simulink model "openMHA_test_db_ar_gaintable"  (R2020b)
settings: Solver=VariableStepAuto  StartTime=0.0  StopTime=stop_time  RelTol=1e-3
InitFcn:
  | initCallback
StopFcn:
  | stopCallback
values from neighbouring files (symbols this model uses):
  buf_a = 65.*ones(num_bands,1)    [test_FFT_to_gain_init.m]    (also in test_db_ar_gaintable_init.m)
  num_bands = 8    [test_FFT_to_gain_init.m]    (also in test_db_ar_gaintable_init.m = 2)
  table_length = length(gtdata)    [test_FFT_to_gain_init.m]    (also in test_db_ar_gaintable_init.m)
  X_high = 93    [test_FFT_to_gain_init.m]    (also in test_db_ar_gaintable_init.m)
undefined symbols (not defined in the file or in its folder): xIn
libraries: dspsrcs4 x13, FPGA_Open_Speech_Tools x4, simulink x4
settings Model: PacingRate=200  Creator=t96f346  LastModifiedBy=wickh

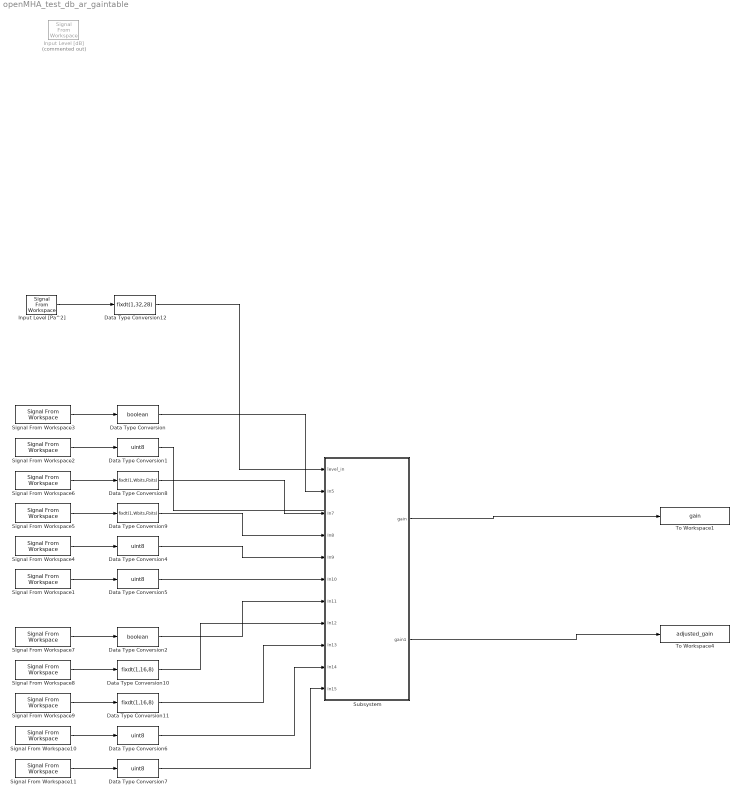
== system openMHA_test_db_ar_gaintable ==
  Data Type Conversion : DataTypeConversion  OutDataTypeStr=boolean
  Data Type Conversion{1,4..7} (5 alike) : DataTypeConversion  OutDataTypeStr=uint8
  Data Type Conversion10 : DataTypeConversion  OutDataTypeStr=fixdt(1,16,8)
  Data Type Conversion11 : DataTypeConversion  OutDataTypeStr=fixdt(1,16,8)
  Data Type Conversion12 : DataTypeConversion  OutDataTypeStr=fixdt(1,32,28)
  Data Type Conversion2 : DataTypeConversion  OutDataTypeStr=boolean
  Data Type Conversion8 : DataTypeConversion  OutDataTypeStr=fixdt(1,Wbits,Fbits)
  Data Type Conversion9 : DataTypeConversion  OutDataTypeStr=fixdt(1,Wbits,Fbits)
  Input Level [Pa^2] : dspsrcs4/Signal From Workspace  X=level_in  Ts=1  nsamps=1  OutputAfterFinalValue=Setting to zero  ignoreOrWarnInputAndFrameLengths=off  OutputFrames=off
  Input Level [dB] : dspsrcs4/Signal From Workspace  Commented=on  X=Lst  Ts=1  nsamps=1  OutputAfterFinalValue=Setting to zero  ignoreOrWarnInputAndFrameLengths=off  OutputFrames=off
  Signal From Workspace1 : dspsrcs4/Signal From Workspace  X=write_addr_r  Ts=1  nsamps=1  OutputAfterFinalValue=Setting to zero  ignoreOrWarnInputAndFrameLengths=off  OutputFrames=off
  Signal From Workspace10 : dspsrcs4/Signal From Workspace  X=write_addr_vy_low  Ts=1  nsamps=1  OutputAfterFinalValue=Setting to zero  ignoreOrWarnInputAndFrameLengths=off  OutputFrames=off
  Signal From Workspace11 : dspsrcs4/Signal From Workspace  X=write_addr_vy_high  Ts=1  nsamps=1  OutputAfterFinalValue=Setting to zero  ignoreOrWarnInputAndFrameLengths=off  OutputFrames=off
  Signal From Workspace2 : dspsrcs4/Signal From Workspace  X=band_num  Ts=1  nsamps=1  OutputAfterFinalValue=Setting to zero  ignoreOrWarnInputAndFrameLengths=off  OutputFrames=off
  Signal From Workspace3 : dspsrcs4/Signal From Workspace  X=write_en_ar  Ts=1  nsamps=1  OutputAfterFinalValue=Setting to zero  ignoreOrWarnInputAndFrameLengths=off  OutputFrames=off
  Signal From Workspace4 : dspsrcs4/Signal From Workspace  X=write_addr_a  Ts=1  nsamps=1  OutputAfterFinalValue=Setting to zero  ignoreOrWarnInputAndFrameLengths=off  OutputFrames=off
  Signal From Workspace5 : dspsrcs4/Signal From Workspace  X=write_data_r  Ts=1  nsamps=1  OutputAfterFinalValue=Setting to zero  ignoreOrWarnInputAndFrameLengths=off  OutputFrames=off
  Signal From Workspace6 : dspsrcs4/Signal From Workspace  X=write_data_a  Ts=1  nsamps=1  OutputAfterFinalValue=Setting to zero  ignoreOrWarnInputAndFrameLengths=off  OutputFrames=off
  Signal From Workspace7 : dspsrcs4/Signal From Workspace  X=write_en_vy  Ts=1  nsamps=1  OutputAfterFinalValue=Setting to zero  ignoreOrWarnInputAndFrameLengths=off  OutputFrames=off
  Signal From Workspace8 : dspsrcs4/Signal From Workspace  X=write_data_vy_low  Ts=1  nsamps=1  OutputAfterFinalValue=Setting to zero  ignoreOrWarnInputAndFrameLengths=off  OutputFrames=off
  Signal From Workspace9 : dspsrcs4/Signal From Workspace  X=write_data_vy_high  Ts=1  nsamps=1  OutputAfterFinalValue=Setting to zero  ignoreOrWarnInputAndFrameLengths=off  OutputFrames=off
  Subsystem : Subsystem
  To Workspace1 : ToWorkspace  VariableName=gain  SampleTime=-1
      settings: Save2DSignal=2-D array (concatenate along first dimension)
  To Workspace4 : ToWorkspace  VariableName=adjusted_gain  SampleTime=-1
      settings: Save2DSignal=2-D array (concatenate along first dimension)
  wires:
  Signal From Workspace2/1 -> Data Type Conversion1/1
  Signal From Workspace3/1 -> Data Type Conversion/1
  Signal From Workspace7/1 -> Data Type Conversion2/1
  Signal From Workspace8/1 -> Data Type Conversion10/1
  Signal From Workspace9/1 -> Data Type Conversion11/1
  Signal From Workspace10/1 -> Data Type Conversion6/1
  Signal From Workspace11/1 -> Data Type Conversion7/1
  Signal From Workspace6/1 -> Data Type Conversion8/1
  Signal From Workspace5/1 -> Data Type Conversion9/1
  Signal From Workspace4/1 -> Data Type Conversion4/1
  Signal From Workspace1/1 -> Data Type Conversion5/1
  Input Level [Pa^2]/1 -> Data Type Conversion12/1
  Data Type Conversion12/1 -> Subsystem/1(level_in)
  Data Type Conversion/1 -> Subsystem/2(In5)
  Data Type Conversion1/1 -> ?
  Data Type Conversion8/1 -> Subsystem/3(In7)
  Data Type Conversion9/1 -> Subsystem/4(In8)
  Data Type Conversion4/1 -> Subsystem/5(In9)
  Data Type Conversion5/1 -> Subsystem/6(In10)
  Data Type Conversion2/1 -> Subsystem/7(In11)
  Data Type Conversion10/1 -> Subsystem/8(In12)
  Data Type Conversion11/1 -> Subsystem/9(In13)
  Data Type Conversion6/1 -> Subsystem/10(In14)
  Data Type Conversion7/1 -> Subsystem/11(In15)
  Subsystem/1(gain) -> To Workspace1/1
  Subsystem/2(gain1) -> To Workspace4/1

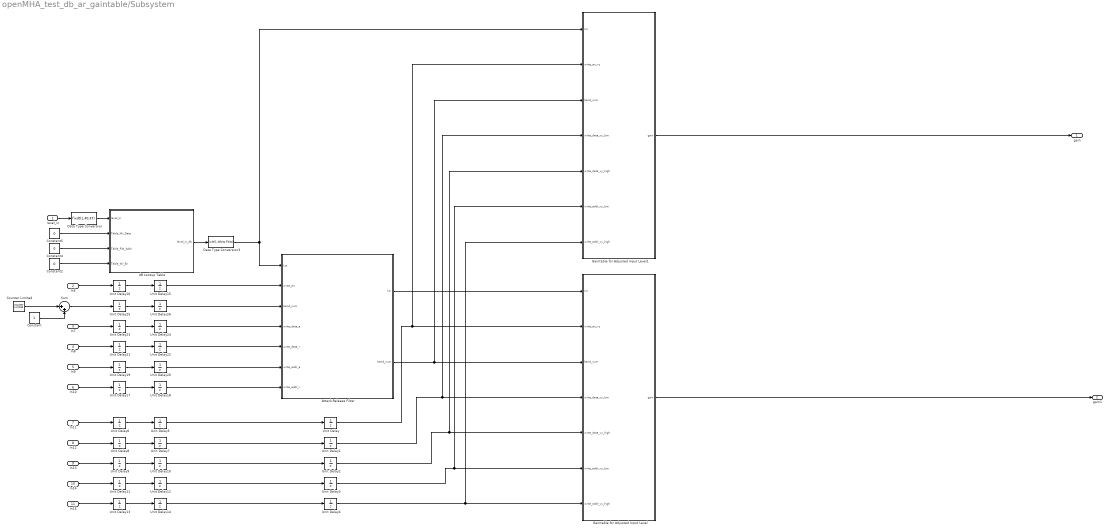
== system openMHA_test_db_ar_gaintable/Subsystem ==
  level_in : Inport
  In5 : Inport  Port=2
  In7 : Inport  Port=3
  In8 : Inport  Port=4
  In9 : Inport  Port=5
  In10 : Inport  Port=6
  In11 : Inport  Port=7
  In12 : Inport  Port=8
  In13 : Inport  Port=9
  In14 : Inport  Port=10
  In15 : Inport  Port=11
  Attack-Release Filter : Subsystem
  Constant : Constant
  Constant2 : Constant  Value=0  OutDataTypeStr=boolean  SampleTime=-1
  Constant4 : Constant  Value=0  OutDataTypeStr=uint16  SampleTime=-1
  Constant5 : Constant  Value=0  OutDataTypeStr=fixdt(1,40,32)  SampleTime=-1
  Counter Limited : simulink/Sources/Counter Limited  uplimit=num_bands-1  tsamp=-1
  Data Type Conversion : DataTypeConversion  OutDataTypeStr=fixdt(1,40,37)
  Data Type Conversion3 : DataTypeConversion  OutDataTypeStr=fixdt(1,Wbits,Fbits)
  Gaintable for Adjusted Input Level : Subsystem
  Gaintable for Adjusted Input Level1 : Subsystem
  Sum : Sum  Inputs=|++
  Unit Delay{,1..3,5..12,15..16,19..26} (22 alike) : UnitDelay  SampleTime=-1  HasFrameUpgradeWarning=on
  Unit Delay{4,13..14,17..18} (5 alike) : UnitDelay  InitialCondition=1  SampleTime=-1  HasFrameUpgradeWarning=on
  dB Lookup Table : Subsystem
  gain : Outport
  gain1 : Outport  Port=2
  wires:
  Unit Delay5/1 -> Unit Delay/1
  Unit Delay24/1 -> Attack-Release Filter/4(write_data_a)
  In8/1 -> Unit Delay21/1
  Unit Delay/1 -> Gaintable for Adjusted Input Level1/2(write_en_vy), Gaintable for Adjusted Input Level/2(write_en_vy)
  In12/1 -> Unit Delay8/1
  Unit Delay2/1 -> Gaintable for Adjusted Input Level1/5(write_data_vy_high), Gaintable for Adjusted Input Level/5(write_data_vy_high)
  Data Type Conversion3/1 -> Attack-Release Filter/1(Lst), Gaintable for Adjusted Input Level1/1(Lin)
  Unit Delay4/1 -> Gaintable for Adjusted Input Level1/7(write_addr_vy_high), Gaintable for Adjusted Input Level/7(write_addr_vy_high)
  Unit Delay26/1 -> Attack-Release Filter/3(band_num)
  In10/1 -> Unit Delay17/1
  In9/1 -> Unit Delay19/1
  Unit Delay17/1 -> Unit Delay18/1
  Attack-Release Filter/1(Lin) -> Gaintable for Adjusted Input Level/1(Lin)
  Unit Delay9/1 -> Unit Delay10/1
  Attack-Release Filter/2("band_num ") -> Gaintable for Adjusted Input Level1/3(band_num), Gaintable for Adjusted Input Level/3(band_num)
  Unit Delay1/1 -> Gaintable for Adjusted Input Level1/4(write_data_vy_low), Gaintable for Adjusted Input Level/4(write_data_vy_low)
  In13/1 -> Unit Delay9/1
  Unit Delay13/1 -> Unit Delay14/1
  Unit Delay11/1 -> Unit Delay12/1
  Unit Delay6/1 -> Unit Delay5/1
  Unit Delay12/1 -> Unit Delay3/1
  Constant2/1 -> dB Lookup Table/4(Table_Wr_En)
  Unit Delay10/1 -> Unit Delay2/1
  Unit Delay7/1 -> Unit Delay1/1
  Unit Delay3/1 -> Gaintable for Adjusted Input Level1/6(write_addr_vy_low), Gaintable for Adjusted Input Level/6(write_addr_vy_low)
  Unit Delay15/1 -> Attack-Release Filter/2(write_en)
  In14/1 -> Unit Delay11/1
  Unit Delay20/1 -> Attack-Release Filter/6(write_addr_a)
  dB Lookup Table/1(level_in_db) -> Data Type Conversion3/1
  Unit Delay18/1 -> Attack-Release Filter/7(write_addr_r)
  In5/1 -> Unit Delay16/1
  Unit Delay16/1 -> Unit Delay15/1
  Unit Delay8/1 -> Unit Delay7/1
  In7/1 -> Unit Delay23/1
  Unit Delay19/1 -> Unit Delay20/1
  Sum/1 -> Unit Delay25/1
  Unit Delay21/1 -> Unit Delay22/1
  Unit Delay25/1 -> Unit Delay26/1
  In11/1 -> Unit Delay6/1
  Unit Delay22/1 -> Attack-Release Filter/5(write_data_r)
  Unit Delay23/1 -> Unit Delay24/1
  Gaintable for Adjusted Input Level1/1(gain) -> gain/1
  Unit Delay14/1 -> Unit Delay4/1
  In15/1 -> Unit Delay13/1
  Constant5/1 -> dB Lookup Table/2(Table_Wr_Data)
  Gaintable for Adjusted Input Level/1(gain) -> gain1/1
  Constant4/1 -> dB Lookup Table/3(Table_RW_Addr)
  level_in/1 -> Data Type Conversion/1
  Data Type Conversion/1 -> dB Lookup Table/1(level_in)
  Counter Limited/1 -> Sum/1
  Constant/1 -> Sum/2

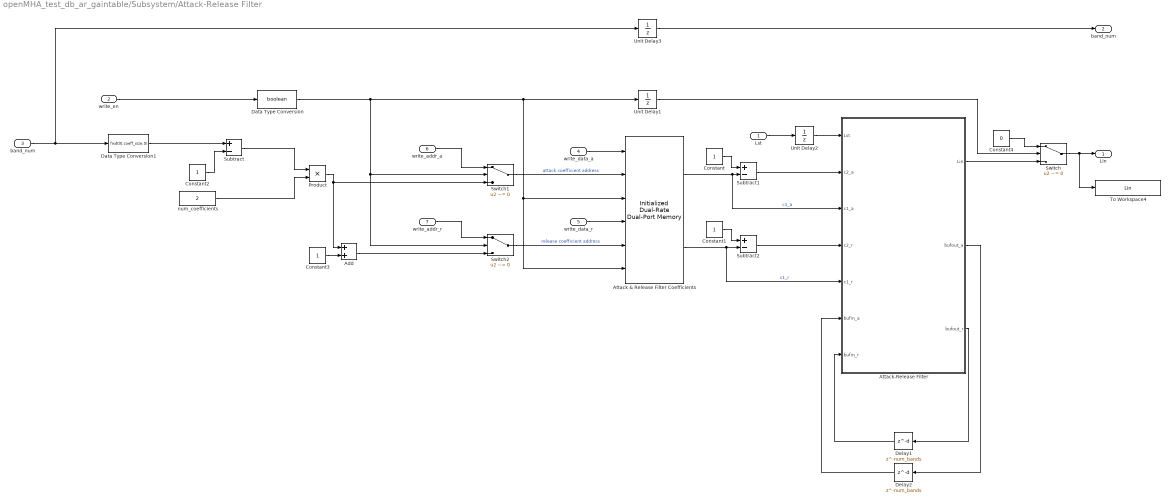
== system openMHA_test_db_ar_gaintable/Subsystem/Attack-Release Filter ==
  Lst : Inport
  write_en : Inport  Port=2
  band_num : Inport  Port=3
  write_data_a : Inport  Port=4
  write_data_r : Inport  Port=5
  write_addr_a : Inport  Port=6
  write_addr_r : Inport  Port=7
  Add : Sum
  Attack & Release Filter Coefficients : FPGA_Open_Speech_Tools/Initialized Dual-Rate Dual-Port Memory  ram_size=coeff_size  Table_Init=ar_coeffs
      settings: SourceProductName=FPGA Open Speech Tools
  Attack-Release Filter : Subsystem
  Constant : Constant  OutDataTypeStr=fixdt(1,Wbits,Fbits)  SampleTime=-1
  Constant1 : Constant  OutDataTypeStr=fixdt(1,Wbits,Fbits)  SampleTime=-1
  Constant2 : Constant  OutDataTypeStr=fixdt(0,coeff_size,0)  SampleTime=-1
  Constant3 : Constant  OutDataTypeStr=uint8  SampleTime=-1
  Constant4 : Constant  Value=0  OutDataTypeStr=fixdt(1,Wbits,Fbits)  SampleTime=-1
  Data Type Conversion : DataTypeConversion  OutDataTypeStr=boolean
  Data Type Conversion1 : DataTypeConversion  OutDataTypeStr=fixdt(0,coeff_size,0)
  Delay1 : Delay  DelayLength=num_bands  InitialCondition=buf_a  UseCircularBuffer=on
  Delay2 : Delay  DelayLength=num_bands  InitialCondition=buf_a  UseCircularBuffer=on
  Product : Product  OutDataTypeStr=fixdt(0,coeff_size,0)
  Subtract : Sum  Inputs=+-  OutDataTypeStr=fixdt(0,coeff_size,0)
  Subtract1 : Sum  Inputs=+-  OutDataTypeStr=fixdt(1,Wbits,Fbits)
  Subtract2 : Sum  Inputs=+-  OutDataTypeStr=fixdt(1,Wbits,Fbits)
  Switch : Switch  Criteria=u2 ~= 0  OutDataTypeStr=fixdt(1,Wbits,Fbits)
  Switch1 : Switch  Criteria=u2 ~= 0  OutDataTypeStr=Inherit: Inherit via back propagation
  Switch2 : Switch  Criteria=u2 ~= 0  OutDataTypeStr=uint8
  To Workspace4 : ToWorkspace  VariableName=Lin  SampleTime=-1
      settings: Save2DSignal=2-D array (concatenate along first dimension)
  Unit Delay1 : UnitDelay  SampleTime=-1  HasFrameUpgradeWarning=on
  Unit Delay2 : UnitDelay  InitialCondition=65  SampleTime=-1  HasFrameUpgradeWarning=on
  Unit Delay3 : UnitDelay  SampleTime=-1  HasFrameUpgradeWarning=on
  num_coefficients : Constant  Value=2  OutDataTypeStr=uint8  SampleTime=-1
  Lin : Outport
  "band_num " : Outport  Port=2
  wires:
  Delay2/1 -> Attack-Release Filter/6(bufin_a)
  write_data_a/1 -> Attack & Release Filter Coefficients/1
  Switch1/1 -> Attack & Release Filter Coefficients/2  "attack coefficient address"
  Switch2/1 -> Attack & Release Filter Coefficients/5  "release coefficient address"
  write_data_r/1 -> Attack & Release Filter Coefficients/4
  Attack-Release Filter/3(bufout_r) -> Delay1/1
  Unit Delay2/1 -> Attack-Release Filter/1(Lst)
  Unit Delay1/1 -> Switch/2
  Lst/1 -> Unit Delay2/1
  Constant1/1 -> Subtract2/1
  Constant/1 -> Subtract1/1
  Switch/1 -> To Workspace4/1, Lin/1
  Attack-Release Filter/1(Lin) -> Switch/3
  Attack-Release Filter/2(bufout_a) -> Delay2/1
  Data Type Conversion/1 -> Unit Delay1/1, Attack & Release Filter Coefficients/3, Attack & Release Filter Coefficients/6, Switch1/2, Switch2/2
  band_num/1 -> Unit Delay3/1, Data Type Conversion1/1
  Constant4/1 -> Switch/1
  write_addr_r/1 -> Switch2/1
  write_en/1 -> Data Type Conversion/1
  Product/1 -> Switch1/3, Add/1
  Delay1/1 -> Attack-Release Filter/7(bufin_r)
  Constant3/1 -> Add/2
  Subtract2/1 -> Attack-Release Filter/4(c2_r)
  Data Type Conversion1/1 -> Subtract/1
  Subtract1/1 -> Attack-Release Filter/2(c2_a)
  write_addr_a/1 -> Switch1/1
  Subtract/1 -> Product/1
  num_coefficients/1 -> Product/2
  Attack & Release Filter Coefficients/2 -> Attack-Release Filter/5(c1_r), Subtract2/2  "c1_r"
  Constant2/1 -> Subtract/2
  Add/1 -> Switch2/3
  Attack & Release Filter Coefficients/1 -> Attack-Release Filter/3(c1_a), Subtract1/2  "c1_a"
  Unit Delay3/1 -> "band_num "/1

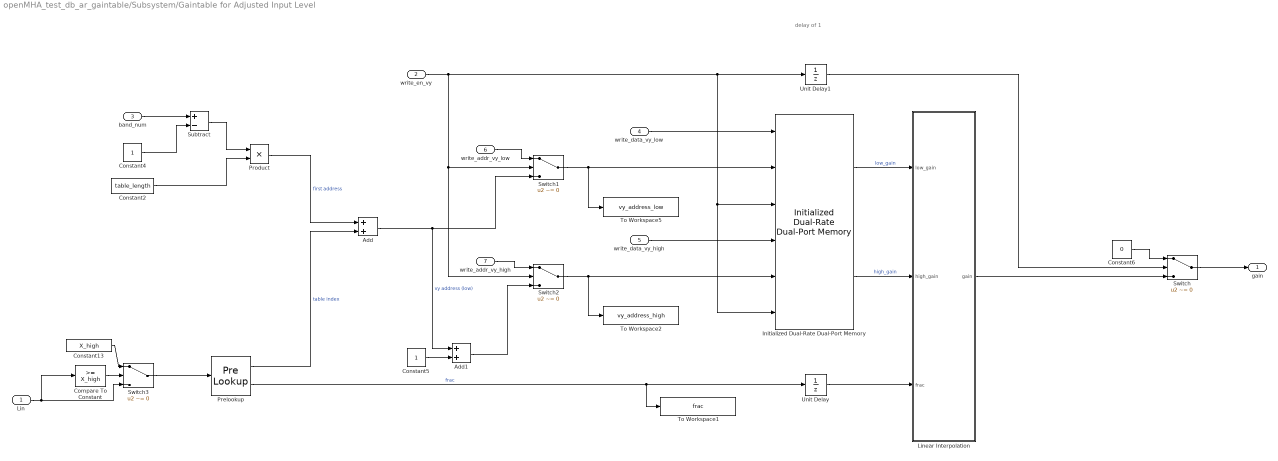
== system openMHA_test_db_ar_gaintable/Subsystem/Gaintable for Adjusted Input Level ==
  note: delay of 1
  Lin : Inport
  write_en_vy : Inport  Port=2
  band_num : Inport  Port=3
  write_data_vy_low : Inport  Port=4
  write_data_vy_high : Inport  Port=5
  write_addr_vy_low : Inport  Port=6
  write_addr_vy_high : Inport  Port=7
  Add : Sum  OutDataTypeStr=uint8
  Add1 : Sum  OutDataTypeStr=uint8
  Compare To Constant : simulink/Logic and Bit Operations/Compare To Constant  relop=>=  const=X_high  OutDataTypeStr=boolean
  Constant13 : Constant  Value=X_high  OutDataTypeStr=fixdt(1,Wbits, Fbits)  SampleTime=-1
  Constant2 : Constant  Value=table_length  OutDataTypeStr=uint8  SampleTime=-1
  Constant4 : Constant  OutDataTypeStr=uint8  SampleTime=-1
  Constant5 : Constant  OutDataTypeStr=uint8  SampleTime=-1
  Constant6 : Constant  Value=0  OutDataTypeStr=fixdt(1,16,8)  SampleTime=-1
  Initialized Dual-Rate Dual-Port Memory : FPGA_Open_Speech_Tools/Initialized Dual-Rate Dual-Port Memory  ram_size=RAM_size  Table_Init=vy
      settings: SourceProductName=FPGA Open Speech Tools
  Linear Interpolation : Subsystem
  Prelookup : PreLookup  BreakpointsData=input_levels_db  IndexSearchMethod=Evenly spaced points  UseLastBreakpoint=on  DiagnosticForOutOfRangeInput=Error  IndexDataTypeStr=uint8
  Product : Product  OutDataTypeStr=Inherit: Same as first input
  Subtract : Sum  Inputs=+-
  Switch : Switch  Criteria=u2 ~= 0  OutDataTypeStr=fixdt(1,16,8)
  Switch1 : Switch  Criteria=u2 ~= 0  OutDataTypeStr=uint8
  Switch2 : Switch  Criteria=u2 ~= 0  OutDataTypeStr=uint8
  Switch3 : Switch  Criteria=u2 ~= 0
  To Workspace1 : ToWorkspace  VariableName=frac  SampleTime=-1
      settings: Save2DSignal=2-D array (concatenate along first dimension)
  To Workspace2 : ToWorkspace  VariableName=vy_address_high  SampleTime=-1
      settings: Save2DSignal=2-D array (concatenate along first dimension)
  To Workspace5 : ToWorkspace  VariableName=vy_address_low  SampleTime=-1
      settings: Save2DSignal=2-D array (concatenate along first dimension)
  Unit Delay : UnitDelay  SampleTime=-1  HasFrameUpgradeWarning=on
  Unit Delay1 : UnitDelay  InitialCondition=1  SampleTime=-1  HasFrameUpgradeWarning=on
  gain : Outport
  wires:
  write_data_vy_low/1 -> Initialized Dual-Rate Dual-Port Memory/1
  Unit Delay/1 -> Linear Interpolation/3(frac)
  Unit Delay1/1 -> Switch/2
  Compare To Constant/1 -> Switch3/2
  Switch/1 -> gain/1
  band_num/1 -> Subtract/1
  Constant6/1 -> Switch/1
  Add/1 -> Switch1/3, Add1/1  "vy address (low)"
  Linear Interpolation/1(gain) -> Switch/3
  Initialized Dual-Rate Dual-Port Memory/2 -> Linear Interpolation/2(high_gain)  "high_gain"
  Switch1/1 -> Initialized Dual-Rate Dual-Port Memory/2, To Workspace5/1
  write_en_vy/1 -> Initialized Dual-Rate Dual-Port Memory/3, Initialized Dual-Rate Dual-Port Memory/6, Unit Delay1/1, Switch1/2, Switch2/2
  Constant5/1 -> Add1/2
  Prelookup/1 -> Add/2  "table index"
  Constant13/1 -> Switch3/1
  Add1/1 -> Switch2/3
  Initialized Dual-Rate Dual-Port Memory/1 -> Linear Interpolation/1(low_gain)  "low_gain"
  Switch2/1 -> Initialized Dual-Rate Dual-Port Memory/5, To Workspace2/1
  Constant4/1 -> Subtract/2
  write_data_vy_high/1 -> Initialized Dual-Rate Dual-Port Memory/4
  Prelookup/2 -> To Workspace1/1, Unit Delay/1  "frac"
  Product/1 -> Add/1  "first address"
  Subtract/1 -> Product/1
  Lin/1 -> Compare To Constant/1, Switch3/3
  Constant2/1 -> Product/2
  Switch3/1 -> Prelookup/1
  write_addr_vy_low/1 -> Switch1/1
  write_addr_vy_high/1 -> Switch2/1

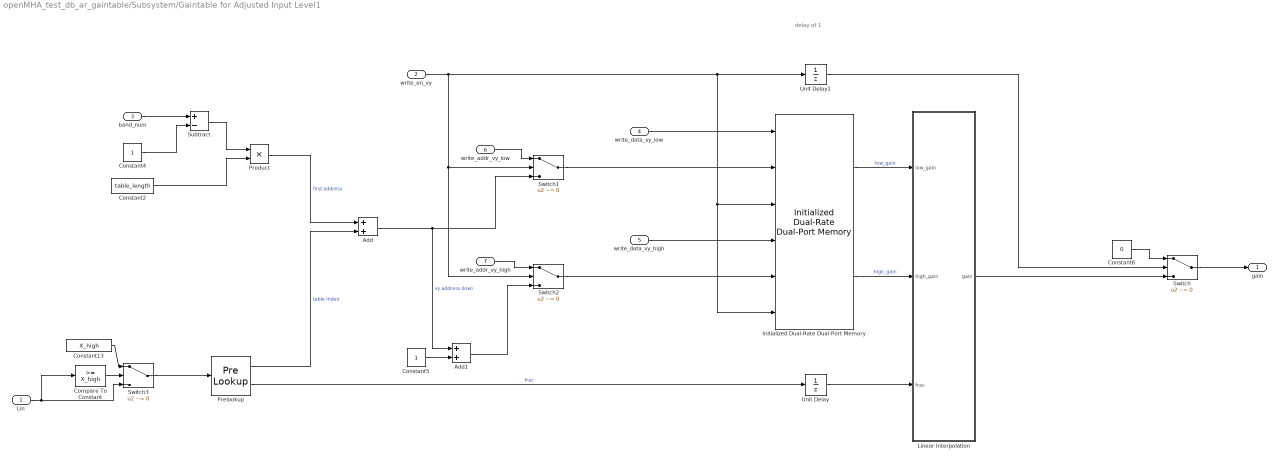
== system openMHA_test_db_ar_gaintable/Subsystem/Gaintable for Adjusted Input Level1 ==
  note: delay of 1
  Lin : Inport
  write_en_vy : Inport  Port=2
  band_num : Inport  Port=3
  write_data_vy_low : Inport  Port=4
  write_data_vy_high : Inport  Port=5
  write_addr_vy_low : Inport  Port=6
  write_addr_vy_high : Inport  Port=7
  Add : Sum  OutDataTypeStr=uint8
  Add1 : Sum  OutDataTypeStr=uint8
  Compare To Constant : simulink/Logic and Bit Operations/Compare To Constant  relop=>=  const=X_high  OutDataTypeStr=boolean
  Constant13 : Constant  Value=X_high  OutDataTypeStr=fixdt(1,Wbits, Fbits)  SampleTime=-1
  Constant2 : Constant  Value=table_length  OutDataTypeStr=uint8  SampleTime=-1
  Constant4 : Constant  OutDataTypeStr=uint8  SampleTime=-1
  Constant5 : Constant  OutDataTypeStr=uint8  SampleTime=-1
  Constant6 : Constant  Value=0  OutDataTypeStr=fixdt(1,16,8)  SampleTime=-1
  Initialized Dual-Rate Dual-Port Memory : FPGA_Open_Speech_Tools/Initialized Dual-Rate Dual-Port Memory  ram_size=RAM_size  Table_Init=vy
      settings: SourceProductName=FPGA Open Speech Tools
  Linear Interpolation : Subsystem
  Prelookup : PreLookup  BreakpointsData=input_levels_db  IndexSearchMethod=Evenly spaced points  UseLastBreakpoint=on  DiagnosticForOutOfRangeInput=Error  IndexDataTypeStr=uint8
  Product : Product  OutDataTypeStr=Inherit: Same as first input
  Subtract : Sum  Inputs=+-
  Switch : Switch  Criteria=u2 ~= 0  OutDataTypeStr=fixdt(1,16,8)
  Switch1 : Switch  Criteria=u2 ~= 0  OutDataTypeStr=uint8
  Switch2 : Switch  Criteria=u2 ~= 0  OutDataTypeStr=uint8
  Switch3 : Switch  Criteria=u2 ~= 0
  Unit Delay : UnitDelay  SampleTime=-1  HasFrameUpgradeWarning=on
  Unit Delay1 : UnitDelay  InitialCondition=1  SampleTime=-1  HasFrameUpgradeWarning=on
  gain : Outport
  wires:
  write_data_vy_low/1 -> Initialized Dual-Rate Dual-Port Memory/1
  Unit Delay/1 -> Linear Interpolation/3(frac)
  Unit Delay1/1 -> Switch/2
  Compare To Constant/1 -> Switch3/2
  Switch/1 -> gain/1
  band_num/1 -> Subtract/1
  Constant6/1 -> Switch/1
  Add/1 -> Switch1/3, Add1/1  "vy address (low)"
  Linear Interpolation/1(gain) -> Switch/3
  Initialized Dual-Rate Dual-Port Memory/2 -> Linear Interpolation/2(high_gain)  "high_gain"
  Switch1/1 -> Initialized Dual-Rate Dual-Port Memory/2
  write_en_vy/1 -> Initialized Dual-Rate Dual-Port Memory/3, Initialized Dual-Rate Dual-Port Memory/6, Unit Delay1/1, Switch1/2, Switch2/2
  Constant5/1 -> Add1/2
  Prelookup/1 -> Add/2  "table index"
  Constant13/1 -> Switch3/1
  Add1/1 -> Switch2/3
  Initialized Dual-Rate Dual-Port Memory/1 -> Linear Interpolation/1(low_gain)  "low_gain"
  Switch2/1 -> Initialized Dual-Rate Dual-Port Memory/5
  Constant4/1 -> Subtract/2
  write_data_vy_high/1 -> Initialized Dual-Rate Dual-Port Memory/4
  Prelookup/2 -> Unit Delay/1  "frac"
  Product/1 -> Add/1  "first address"
  Subtract/1 -> Product/1
  Lin/1 -> Compare To Constant/1, Switch3/3
  Constant2/1 -> Product/2
  Switch3/1 -> Prelookup/1
  write_addr_vy_low/1 -> Switch1/1
  write_addr_vy_high/1 -> Switch2/1

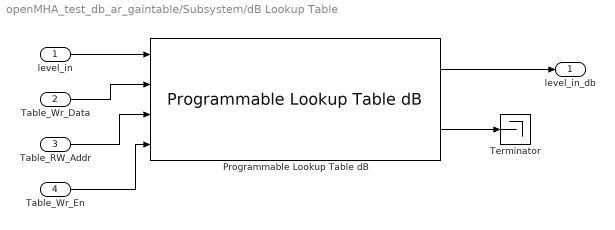
== system openMHA_test_db_ar_gaintable/Subsystem/dB Lookup Table ==
  level_in : Inport
  Table_Wr_Data : Inport  Port=2
  Table_RW_Addr : Inport  Port=3
  Table_Wr_En : Inport  Port=4
  Programmable Lookup Table dB : FPGA_Open_Speech_Tools/Programmable Lookup Table dB  tableFnParam=10.*log10(2500000000.*xIn)  SAVE_TABLE=off  maxInput=1  floorParam=2^-31  errorParam=1  ERR_DIAG=on  PLOT_TABLE=off  nBitsParam=5  mBitsParam=4  IGOTTHIS=off  W_bits=40  F_bits=37  tableInit=0  binaryOffset=0
      link override High_LUT/ram_data: InitialCondition=55.36
      link override Linear_Approximation/Unit Delay: InitialCondition=65
      link override LogAddressing/Delay1: InitialCondition=13
      link override LogAddressing/Delay2: InitialCondition=0.0001265
      link override Low_LUT/ram_data: InitialCondition=54.85
      link override Unit Delay1: InitialCondition=0.0001265
      link override Unit Delay2: InitialCondition=0.0001265
      link override Unit Delay3: InitialCondition=144
      settings: SourceProductName=FPGA Open Speech Tools
  Terminator : Terminator
  level_in_db : Outport
  wires:
  Programmable Lookup Table dB/2 -> Terminator/1
  level_in/1 -> Programmable Lookup Table dB/1
  Programmable Lookup Table dB/1 -> level_in_db/1
  Table_Wr_En/1 -> Programmable Lookup Table dB/4
  Table_Wr_Data/1 -> Programmable Lookup Table dB/2
  Table_RW_Addr/1 -> Programmable Lookup Table dB/3

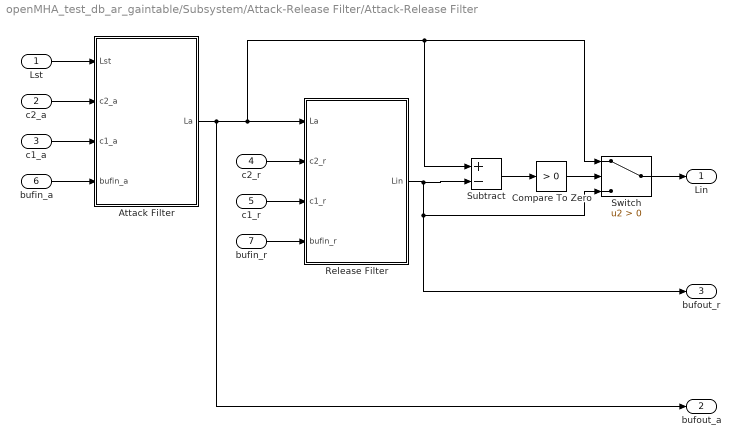
== system openMHA_test_db_ar_gaintable/Subsystem/Attack-Release Filter/Attack-Release Filter ==
  Lst : Inport
  c2_a : Inport  Port=2
  c1_a : Inport  Port=3
  c2_r : Inport  Port=4
  c1_r : Inport  Port=5
  bufin_a : Inport  Port=6
  bufin_r : Inport  Port=7
  Attack Filter : Subsystem  TreatAsAtomicUnit=on
  Compare To Zero : simulink/Logic and Bit Operations/Compare To Zero  relop=>  OutDataTypeStr=boolean
  Release Filter : Subsystem  TreatAsAtomicUnit=on
  Subtract : Sum  Inputs=+-  OutDataTypeStr=fixdt(0,Wbits,Fbits)
  Switch : Switch  Criteria=u2 > Threshold  OutDataTypeStr=fixdt(0,Wbits,Fbits)
  Lin : Outport  VectorParamsAs1DForOutWhenUnconnected=off
  bufout_a : Outport  Port=2  VectorParamsAs1DForOutWhenUnconnected=off
  bufout_r : Outport  Port=3  VectorParamsAs1DForOutWhenUnconnected=off
  wires:
  Lst/1 -> Attack Filter/1(Lst)
  c2_a/1 -> Attack Filter/2(c2_a)
  c1_a/1 -> Attack Filter/3(c1_a)
  bufin_a/1 -> Attack Filter/4(bufin_a)
  c2_r/1 -> Release Filter/2(c2_r)
  c1_r/1 -> Release Filter/3(c1_r)
  bufin_r/1 -> Release Filter/4(bufin_r)
  Attack Filter/1(La) -> bufout_a/1, Switch/1, Subtract/1, Release Filter/1(La)
  Compare To Zero/1 -> Switch/2
  Release Filter/1(Lin) -> Subtract/2, Switch/3, bufout_r/1
  Subtract/1 -> Compare To Zero/1
  Switch/1 -> Lin/1

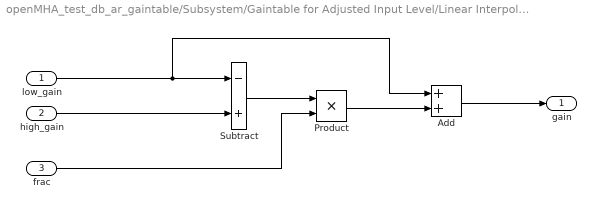
== system openMHA_test_db_ar_gaintable/Subsystem/Gaintable for Adjusted Input Level/Linear Interpolation ==
  low_gain : Inport
  high_gain : Inport  Port=2
  frac : Inport  Port=3
  Add : Sum
  Product : Product  OutDataTypeStr=Inherit: Same as first input
  Subtract : Sum  Inputs=-+
  gain : Outport
  wires:
  high_gain/1 -> Subtract/2
  low_gain/1 -> Add/1, Subtract/1
  Subtract/1 -> Product/1
  frac/1 -> Product/2
  Product/1 -> Add/2
  Add/1 -> gain/1

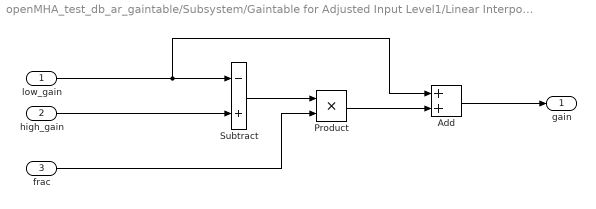
== system openMHA_test_db_ar_gaintable/Subsystem/Gaintable for Adjusted Input Level1/Linear Interpolation ==
  low_gain : Inport
  high_gain : Inport  Port=2
  frac : Inport  Port=3
  Add : Sum
  Product : Product  OutDataTypeStr=Inherit: Same as first input
  Subtract : Sum  Inputs=-+
  gain : Outport
  wires:
  high_gain/1 -> Subtract/2
  low_gain/1 -> Add/1, Subtract/1
  Subtract/1 -> Product/1
  frac/1 -> Product/2
  Product/1 -> Add/2
  Add/1 -> gain/1

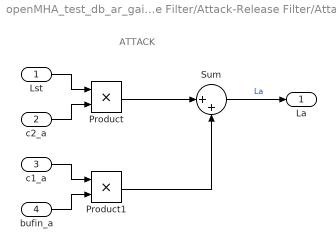
== system openMHA_test_db_ar_gaintable/Subsystem/Attack-Release Filter/Attack-Release Filter/Attack Filter ==
  note: ATTACK
  Lst : Inport
  c2_a : Inport  Port=2
  c1_a : Inport  Port=3
  bufin_a : Inport  Port=4
  Product : Product  OutDataTypeStr=fixdt(0,Wbits,Fbits)
  Product1 : Product  OutDataTypeStr=fixdt(0,Wbits,Fbits)
  Sum : Sum  Inputs=|++  OutDataTypeStr=fixdt(0,Wbits,Fbits)
  La : Outport  InitialOutput=0  VectorParamsAs1DForOutWhenUnconnected=off
  wires:
  Lst/1 -> Product/1
  Product/1 -> Sum/1
  Sum/1 -> La/1  "La"
  bufin_a/1 -> Product1/2
  Product1/1 -> Sum/2
  c2_a/1 -> Product/2
  c1_a/1 -> Product1/1

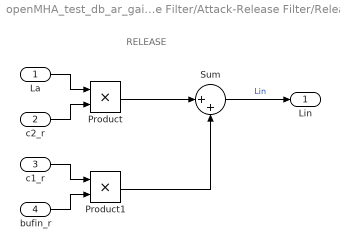
== system openMHA_test_db_ar_gaintable/Subsystem/Attack-Release Filter/Attack-Release Filter/Release Filter ==
  note: RELEASE
  La : Inport
  c2_r : Inport  Port=2
  c1_r : Inport  Port=3
  bufin_r : Inport  Port=4
  Product : Product  OutDataTypeStr=fixdt(0,Wbits,Fbits)
  Product1 : Product  OutDataTypeStr=fixdt(0,Wbits,Fbits)
  Sum : Sum  Inputs=|++  OutDataTypeStr=fixdt(0,Wbits,Fbits)
  Lin : Outport  InitialOutput=0  VectorParamsAs1DForOutWhenUnconnected=off
  wires:
  Sum/1 -> Lin/1  "Lin"
  c2_r/1 -> Product/2
  c1_r/1 -> Product1/1
  La/1 -> Product/1
  Product1/1 -> Sum/2
  Product/1 -> Sum/1
  bufin_r/1 -> Product1/2
